simulink model "prob4"  (R2020b)
settings: Solver=VariableStepAuto  StartTime=0.0  StopTime=10.0  RelTol=1e-3
settings Model: Creator=Nitin  LastModifiedBy=Nitin

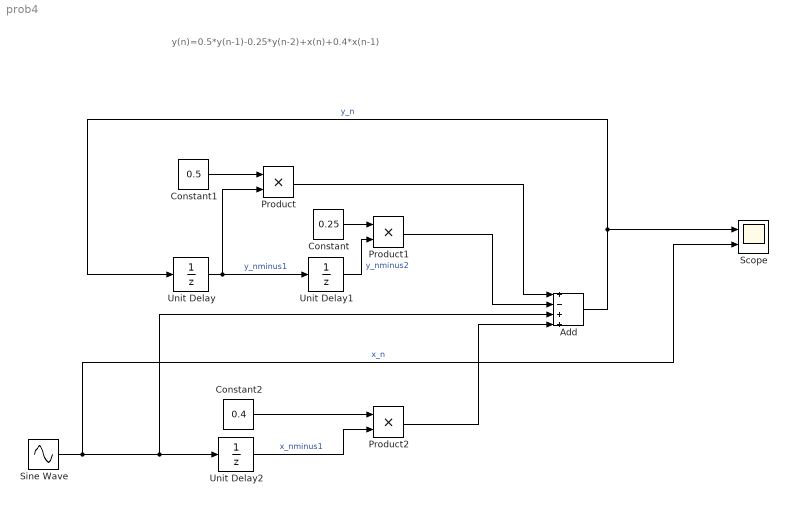
== system prob4 ==
  note: y(n)=0.5*y(n-1)-0.25*y(n-2)+x(n)+0.4*x(n-1)
  Add : Sum  Inputs=+-++
  Constant : Constant  Value=0.25
  Constant1 : Constant  Value=0.5
  Constant2 : Constant  Value=0.4
  Product : Product
  Product1 : Product
  Product2 : Product
  Scope : Scope  NumInputPorts=2
  Sine Wave : Sin  SampleTime=0
  Unit Delay : UnitDelay  SampleTime=-1  HasFrameUpgradeWarning=on
  Unit Delay1 : UnitDelay  SampleTime=-1  HasFrameUpgradeWarning=on
  Unit Delay2 : UnitDelay  SampleTime=-1  HasFrameUpgradeWarning=on
  wires:
  Constant/1 -> Product1/1
  Constant1/1 -> Product/1
  Sine Wave/1 -> Scope/2, Add/3, Unit Delay2/1  "x_n"
  Product/1 -> Add/1
  Constant2/1 -> Product2/1
  Unit Delay2/1 -> Product2/2  "x_nminus1"
  Product1/1 -> Add/2
  Product2/1 -> Add/4
  Add/1 -> Scope/1, Unit Delay/1  "y_n"
  Unit Delay1/1 -> Product1/2  "y_nminus2"
  Unit Delay/1 -> Unit Delay1/1, Product/2  "y_nminus1"
